simulink model "my_macro_1"  (R2026a)
settings: Solver=VariableStepAuto
values from neighbouring files (symbols this model uses):
  A = [A_init, zeros(5,1) ... (first row only)    [IP_MACRO.m]    (also in testes_30_03.m)
  B = [B_init ... (first row only)    [IP_MACRO.m]    (also in testes_30_03.m)
  C = [C_init, zeros(2,1)]    [IP_MACRO.m]    (also in testes_30_03.m)
  D = zeros(2,1)    [IP_MACRO.m]    (also in testes_30_03.m)
undefined symbols (not defined in the file or in its folder): K_q6
settings Model: Creator=sofiaduarte  LastModifiedBy=sofiaduarte

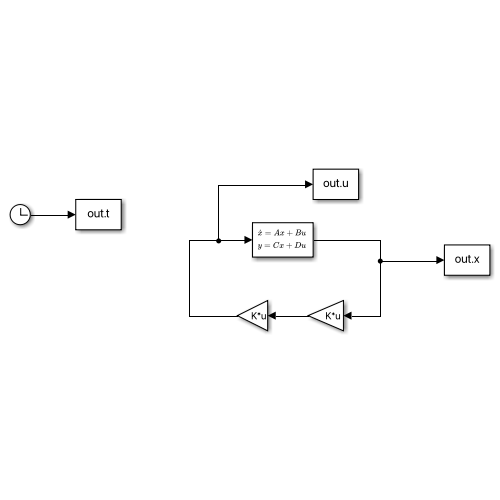
[thumbnail: Simulink's stored preview of the top-level diagram]
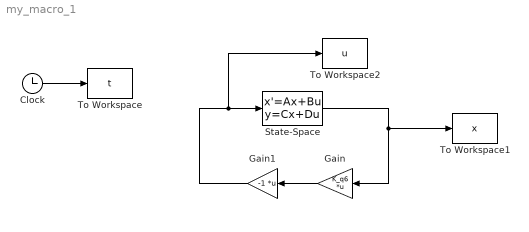
== system my_macro_1 ==
  Clock : Clock
  Gain : Gain  Gain=K_q6  Multiplication=Matrix(K*u)
  Gain1 : Gain  Gain=-1  Multiplication=Matrix(K*u)
  State-Space : StateSpace  A=A  B=B  C=C  D=D  InitialCondition=0
  To Workspace : ToWorkspace  VariableName=t  SaveFormat=Structure With Time  SampleTime=-1
  To Workspace1 : ToWorkspace  VariableName=x  SampleTime=-1
  To Workspace2 : ToWorkspace  VariableName=u  SampleTime=-1
  wires:
  Clock/1 -> To Workspace/1
  Gain1/1 -> To Workspace2/1, State-Space/1
  State-Space/1 -> Gain/1, To Workspace1/1
  Gain/1 -> Gain1/1
